simulink model "SE_1"  (R2024a)
settings: Solver=FixedStepAuto  StartTime=0.0  StopTime=10  RelTol=1e-3
libraries: simulink_extras x4
settings Model: Creator=levm1106  LastModifiedBy=levm1106
settings DebuggingCC: UnconnectedInputMsg=warning  UnconnectedOutputMsg=warning  UnconnectedLineMsg=warning
settings ModelReferenceCC: EnableRefExpFcnMdlSchedulingChecks=on
settings RTWCC: GPUComputeCapability=3.5  DLArmComputeVersion=19.05

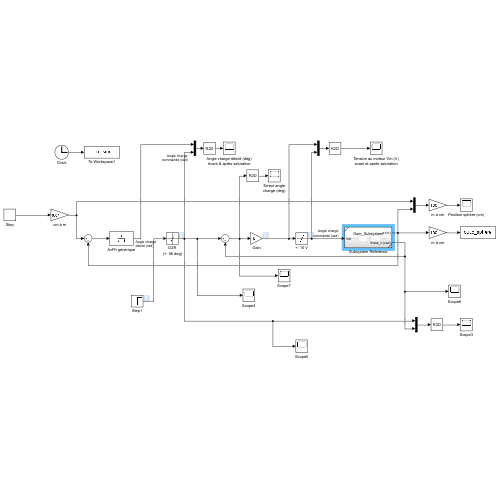
[thumbnail: Simulink's stored preview of the top-level diagram]
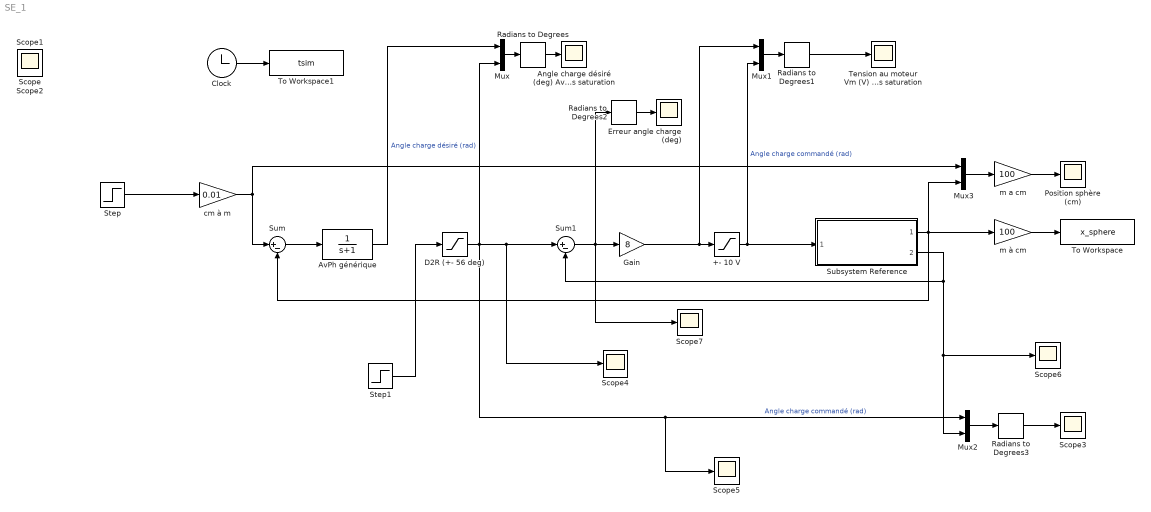
== system SE_1 ==
  +- 10 V : Saturate  UpperLimit=10  LowerLimit=-10
  Angle charge désiré (deg) Avant & après saturation : Scope
  AvPh générique : TransferFcn  Denominator=[1 1]
  Clock : Clock
  D2R (+- 56 deg) : Saturate  UpperLimit=0.9974  LowerLimit=-0.9974
  Erreur angle charge (deg) : Scope
  Gain : Gain  Gain=8
  Mux{,1..3} (4 alike) : Mux  Inputs=2
  Position sphère (cm) : Scope
  Radians to Degrees{,1..3} (4 alike) : simulink_extras/Transformations/Radians to Degrees
  Scope{,1..7} (8 alike) : Scope
  Step : Step  Time=0  Before=1  SampleTime=0
  Step1 : Step  Time=0  Before=pi/6  After=pi/6  SampleTime=0.01
  Subsystem Reference : Subsystem  ReferencedSubsystem=Gsm_Subsystem
  Sum : Sum  Inputs=|+-
  Sum1 : Sum  Inputs=|+-
  Tension au moteur Vm (V) avant et après saturation : Scope
  To Workspace : ToWorkspace  VariableName=x_sphere  SaveFormat=Timeseries  SampleTime=-1
  To Workspace1 : ToWorkspace  VariableName=tsim  SaveFormat=Timeseries  SampleTime=-1
  cm à m : Gain  Gain=0.01
  m a cm : Gain  Gain=100
  m à cm : Gain  Gain=100
  wires:
  Step/1 -> cm à m/1
  Sum/1 -> AvPh générique/1
  cm à m/1 -> Sum/1, Mux3/1
  AvPh générique/1 -> Mux/1  "Angle charge désiré (rad)"
  D2R (+- 56 deg)/1 -> Sum1/1, Scope4/1, Mux/2, Scope5/1, Mux2/1  "Angle charge commandé (rad)"
  Mux/1 -> Radians to Degrees/1
  Radians to Degrees/1 -> Angle charge désiré (deg) Avant & après saturation/1
  Gain/1 -> Mux1/1, +- 10 V/1
  Mux1/1 -> Radians to Degrees1/1
  Radians to Degrees1/1 -> Tension au moteur Vm (V) avant et après saturation/1
  +- 10 V/1 -> Subsystem Reference/1, Mux1/2  "Angle charge commandé (rad)"
  Radians to Degrees2/1 -> Erreur angle charge (deg)/1
  Subsystem Reference/1 -> Mux3/2, m à cm/1, Sum/2
  m à cm/1 -> To Workspace/1
  Mux2/1 -> Radians to Degrees3/1
  Radians to Degrees3/1 -> Scope3/1
  Subsystem Reference/2 -> Sum1/2, Mux2/2, Scope6/1
  Mux3/1 -> m a cm/1
  m a cm/1 -> Position sphère (cm)/1
  Clock/1 -> To Workspace1/1
  Sum1/1 -> Radians to Degrees2/1, Scope7/1, Gain/1
  Step1/1 -> D2R (+- 56 deg)/1
